simulink model "plant"  (R2022a)
settings: Solver=VariableStepAuto  StartTime=0.0  StopTime=10.0  RelTol=1e-3
settings Model: Creator=Parsa Noori  LastModifiedBy=Parsa Noori

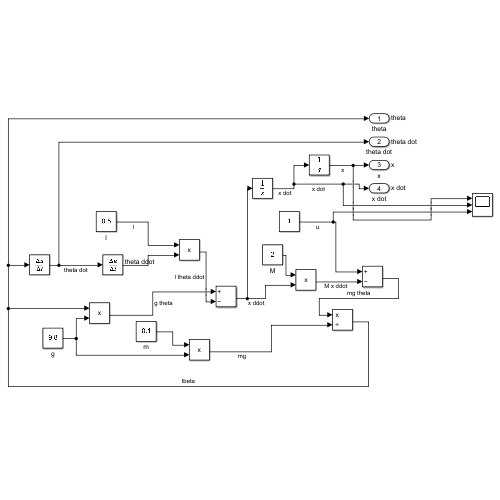
[thumbnail: Simulink's stored preview of the top-level diagram]
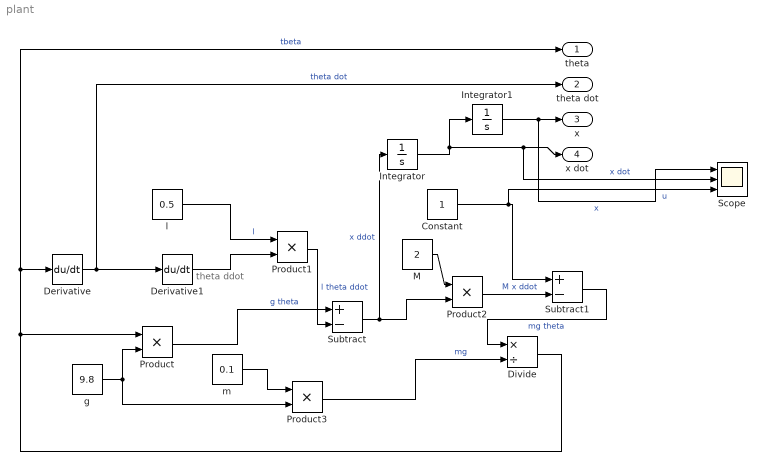
== system plant ==
  note: theta ddot
  Constant : Constant
  Derivative : Derivative
  Derivative1 : Derivative
  Divide : Product  Inputs=*/
  Integrator : Integrator
  Integrator1 : Integrator
  M : Constant  Value=2
  Product{,1..3} (4 alike) : Product
  Scope : Scope  NumInputPorts=3
  Subtract : Sum  Inputs=+-
  Subtract1 : Sum  Inputs=+-
  g : Constant  Value=9.8
  l : Constant  Value=0.5
  m : Constant  Value=0.1
  theta : Outport  SignalName=theta
  theta dot : Outport  Port=2  SignalName=theta dot
  x : Outport  Port=3  SignalName=x
  x dot : Outport  Port=4  SignalName=x dot
  wires:
  g/1 -> Product3/2, Product/2
  l/1 -> Product1/1  "l"
  Derivative/1 -> theta dot/1, Derivative1/1  "theta dot"
  Derivative1/1 -> Product1/2
  Product1/1 -> Subtract/2  "l theta ddot"
  Subtract/1 -> Integrator/1, Product2/2  "x ddot"
  Product/1 -> Subtract/1  "g theta"
  M/1 -> Product2/1
  Product2/1 -> Subtract1/2  "M x ddot"
  Subtract1/1 -> Divide/1  "mg theta"
  m/1 -> Product3/1
  Product3/1 -> Divide/2  "mg"
  Divide/1 -> Product/1, theta/1, Derivative/1  "tbeta"
  Integrator/1 -> Integrator1/1, Scope/2, x dot/1  "x dot"
  Integrator1/1 -> Scope/1, x/1  "x"
  Constant/1 -> Scope/3, Subtract1/1  "u"
